simulink model "MPC_fmincon"  (R2023a)
settings: Solver=ode1  StartTime=0.0  StopTime=inf  FixedStep=0.002  RelTol=1e-3  EnableMultiTasking=on
undefined symbols (not defined in the file): HIL
libraries: quarc_library x18, simulink x1
settings Model: ExtModeTrigDuration=10000  Creator=bajdus  LastModifiedBy=pindiche
settings SolverCC: AlgebraicLoopSolver=TrustRegion  PositivePriorityOrder=on
settings DataIOCC: ReturnWorkspaceOutputs=off
settings DebuggingCC: UnconnectedInputMsg=warning  UnconnectedOutputMsg=warning  UnconnectedLineMsg=warning  ArithmeticOperatorsInVariantConditions=warning
settings HardwareCC: ProdBitPerLong=64  ProdLargestAtomicInteger=LongLong  ProdLargestAtomicFloat=Double  ProdLongLongMode=on  ProdHWDeviceType=ARM Compatible->ARM 64-bit (LP64)
settings ModelReferenceCC: EnableRefExpFcnMdlSchedulingChecks=on
settings SFSimCC: SimUseLocalCustomCode=off  CustomCodeUndefinedFunction=UseInterfaceOnly
settings RTWCC: Description=QUARC Linux QCar2 Target Using Toolchain  SystemTargetFile=quarc_linux_qcar2.tlc  TemplateMakefile=quarc_default_tmf  RTWUseLocalCustomCode=off  Toolchain=QUARC linux_qcar2 | gmake (64-bit Windows)  BuildConfiguration=Faster Runs
settings CodeAppCC: StateflowObjectComments=on
settings STFCustomTargetCC: SystemTargetFile=quarc_linux_qcar2.tlc
settings GRTTargetCC: ParMdlRefBuildCompliant=off  CompOptLevelCompliant=off  CombineOutputUpdateFcns=off  MatFileLogging=off  CPPClassGenCompliant=off  GRTInterface=on  ExtMode=on  ExtModeMexFile=quarc_comm  ExtModeMexArgs='-w -d /tmp -uri %u', 'tcpip://192.168.1.126:17001'
settings ConfigComp: CovMetricSettings=dswe

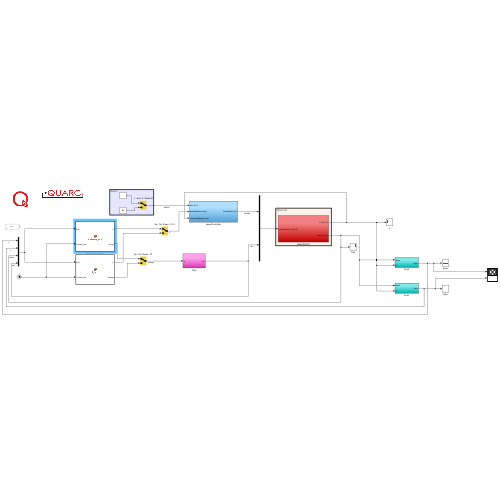
[thumbnail: Simulink's stored preview of the top-level diagram]
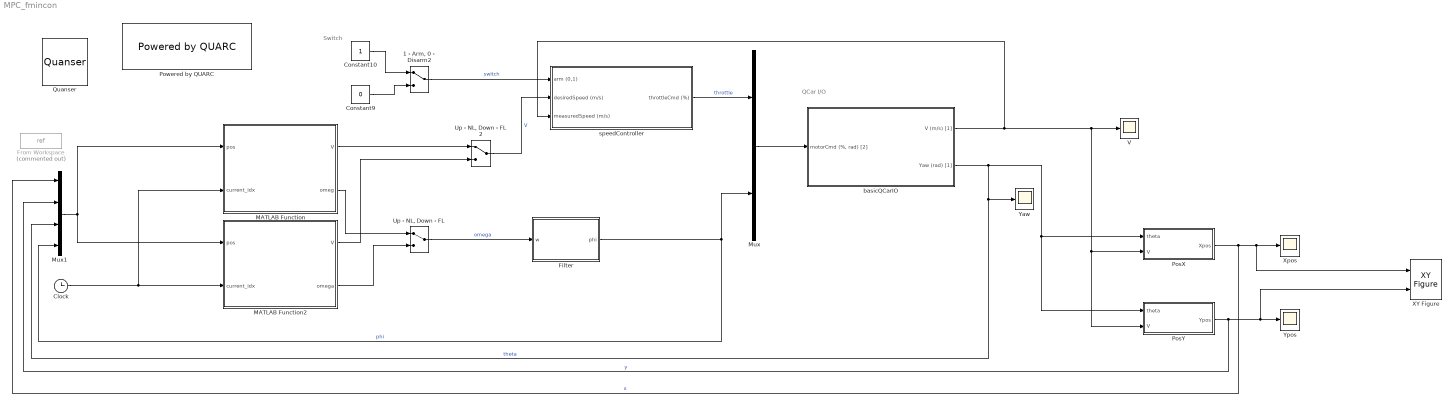
== system MPC_fmincon ==
  note: QCar I/O
  note: Switch
  "1 - Arm, 0 - Disarm2" : ManualSwitch
  Clock : Clock
  Constant10 : Constant
  Constant9 : Constant  Value=0
  Filter : Subsystem
  From Workspace : FromWorkspace  Commented=on  VariableName=ref
  MATLAB Function : MATLAB Function  TreatAsAtomicUnit=on
  MATLAB Function2 : MATLAB Function  TreatAsAtomicUnit=on
  Mux : Mux  Inputs=2
  Mux1 : Mux
  PosX : Subsystem
  PosY : Subsystem
  Powered by QUARC : quarc_library/Logos/Powered by QUARC
  Quanser : quarc_library/Logos/Quanser
  "Up - NL, Down - FL" : ManualSwitch
  "Up - NL, Down - FL 2" : ManualSwitch
  V : Scope
  XY Figure : quarc_library/Sinks/Figures/XY Figure  figure_mode=Use figure window  figure_tag=figure1  axes_tag=axes1  plot_mode=Time-based  minimum_x=-5  maximum_x=5  minimum_y=-5  maximum_y=5  buffer_size=1000000  update_rate=100  initial_position="1.8          41.8         439.2         331.2"  initial_visibility=off  sample_time=-1
      settings: SourceProductName=QUARC Targets
  Xpos : Scope
  Yaw : Scope
  Ypos : Scope
  basicQCarIO : Subsystem
  speedController : Subsystem
  wires:
  Mux/1 -> basicQCarIO/1("motorCmd (%, rad) [2]")
  "1 - Arm, 0 - Disarm2"/1 -> speedController/1(arm (0,1))  "switch"
  Constant10/1 -> "1 - Arm, 0 - Disarm2"/1
  speedController/1(throttleCmd (%)) -> Mux/1  "throttle"
  basicQCarIO/1(V (m/s) [1]) -> speedController/3(measuredSpeed (m/s)), V/1, PosX/2(V), PosY/2(V)
  Constant9/1 -> "1 - Arm, 0 - Disarm2"/2
  PosX/1(Xpos) -> XY Figure/1, Xpos/1, Mux1/1  "x"
  PosY/1(Ypos) -> XY Figure/2, Ypos/1, Mux1/2  "y"
  basicQCarIO/2(Yaw (rad) [1]) -> Mux1/3, Yaw/1, PosY/1(theta), PosX/1(theta)  "theta"
  Filter/1(phi) -> Mux1/4, Mux/2  "phi"
  MATLAB Function/1(V) -> "Up - NL, Down - FL 2"/1
  MATLAB Function2/1(V) -> "Up - NL, Down - FL 2"/2
  "Up - NL, Down - FL 2"/1 -> speedController/2(desiredSpeed (m/s))  "V"
  MATLAB Function/2(omeg) -> "Up - NL, Down - FL"/1
  MATLAB Function2/2(omega) -> "Up - NL, Down - FL"/2
  Mux1/1 -> MATLAB Function/1(pos), MATLAB Function2/1(pos)
  Clock/1 -> MATLAB Function/2(current_idx), MATLAB Function2/2(current_idx)
  "Up - NL, Down - FL"/1 -> Filter/1(w)  "omega"

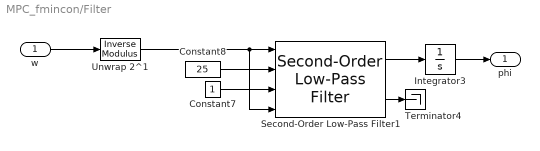
== system MPC_fmincon/Filter ==
  w : Inport
  Constant7 : Constant
  Constant8 : Constant  Value=25
  Integrator3 : Integrator
  Second-Order Low-Pass Filter1 : quarc_library/Continuous/Second-Order Low-Pass Filter  params_source=External (input ports)  input_width=1  input_zeta=1  input_init=0
  Terminator4 : Terminator
  Unwrap 2^1 : quarc_library/Discontinuities/Inverse Modulus  modulus=16777215  output_derivative=off  output_revolutions=off  max_x=Inf  min_x=-Inf
  phi : Outport
  wires:
  Constant8/1 -> Second-Order Low-Pass Filter1/2
  Constant7/1 -> Second-Order Low-Pass Filter1/3
  Second-Order Low-Pass Filter1/1 -> Integrator3/1
  Unwrap 2^1/1 -> Second-Order Low-Pass Filter1/4, Second-Order Low-Pass Filter1/1
  w/1 -> Unwrap 2^1/1
  Second-Order Low-Pass Filter1/2 -> Terminator4/1
  Integrator3/1 -> phi/1

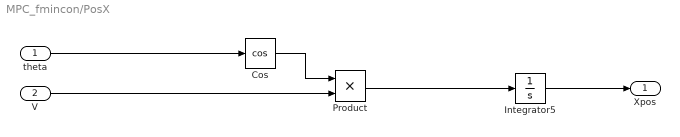
== system MPC_fmincon/PosX ==
  theta : Inport
  V : Inport  Port=2
  Cos : Trigonometry  Operator=cos
  Integrator5 : Integrator
  Product : Product
  Xpos : Outport
  wires:
  Cos/1 -> Product/1
  theta/1 -> Cos/1
  V/1 -> Product/2
  Integrator5/1 -> Xpos/1
  Product/1 -> Integrator5/1

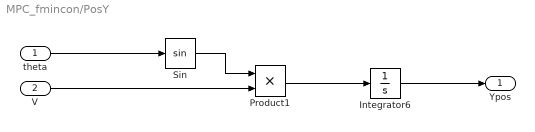
== system MPC_fmincon/PosY ==
  theta : Inport
  V : Inport  Port=2
  Integrator6 : Integrator
  Product1 : Product
  Sin : Trigonometry
  Ypos : Outport
  wires:
  theta/1 -> Sin/1
  V/1 -> Product1/2
  Sin/1 -> Product1/1
  Integrator6/1 -> Ypos/1
  Product1/1 -> Integrator6/1

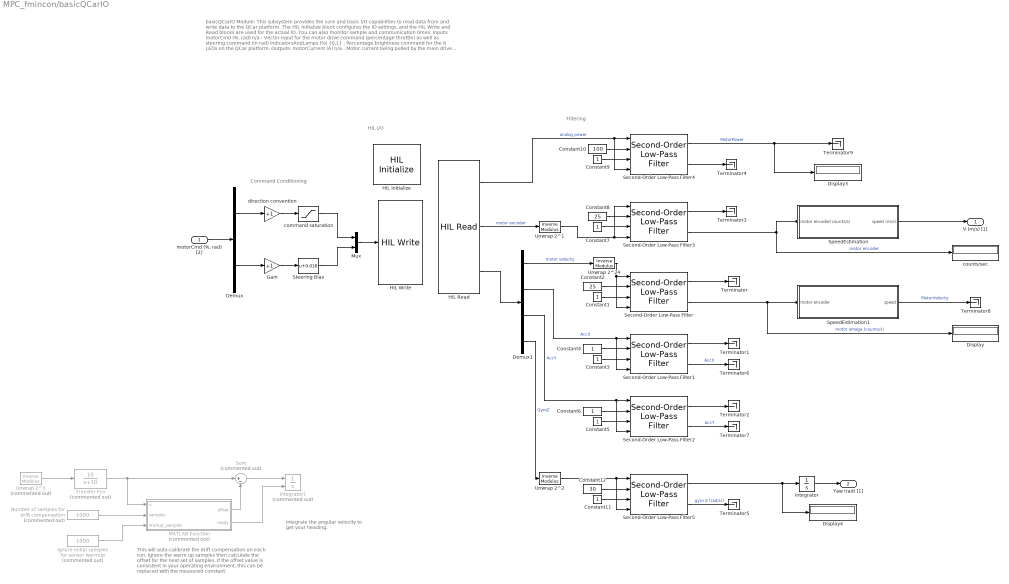
== system MPC_fmincon/basicQCarIO ==
  note: Filtering
  note: basicQCarIO Module:
      |
      | This subsystem provides the core and basic I/O capabilities to read data from and write data to the QCar platform. The HIL Initialize block configures the IO settings, and the HIL Write and Read blocks are used for the actual IO. You can also monitor sample and communication times.
      |
      | Inputs:
      | motorCmd (%, rad) n/a : Vector input for the motor drive command (percentage throttle) as well as steering command (in rad)
      | indicatorsAndLamps (%) {0,1} : Percentage brightness command for the 8 LEDs on the QCar platform.
      |
      | Outputs:
      | motorCurrent (A) n/a : Motor current being pulled by the main drive motor
      | batteryVoltage (V) {0, 12.6} : Current battery voltage reading
      | motorSpeed (counts/s) n/a : Drive motor speed measured using an encoder (do not confuse with wheel speed as this measurement is at the drive shaft)
  note: Command Conditioning
  note: HIL I/O
  note: Integrate the angular velocity to
      | get your heading.
  note: This will auto-calibrate the drift compensation
      | on each run. Ignore the warm up samples
      | then calculate the offset for the next set of samples.
      | If the offset value is consistent in your operating
      | environment, this can be replaced with the measured
      | constant.
  "motorCmd (%, rad) [2]" : Inport
  Constant{1,3..7,9,11} (8 alike) : Constant
  Constant10 : Constant  Value=100
  Constant12 : Constant  Value=30
  Constant2 : Constant  Value=25
  Constant8 : Constant  Value=25
  Demux : Demux  Outputs=2
  Demux1 : Demux
  Display : Display
  Display3 : Display
  Display4 : Display
  Gain : Gain  Gain=+1
  HIL Initialize : quarc_library/Data Acquisition/Generic/Configuration/HIL Initialize  object_name=HIL-2  board_type=qcar2  board_number=0  board_options=gyro_fs=250;gyro_rate=500;gyro_bw=125;gyro_ord=3;accel_fs=16;accel_rate=1000;accel_bw=250;accel_ord=3;temp_bw=4000;enc0_dir=0;enc1_dir=0;enc2_dir=0;steer_bias=0.05;  exclusive=off  active=on  hardware_clocks=[]  clock_modes=[]  initial_clock_frequencies=[]  set_clock_params_at_start=off  set_clock_params_at_switch_in=off  set_clock_frequencies_at_start=off  set_clock_frequencies_at_switch_in=off  analog_input_channels=[0:4]  analog_input_configurations=[]  analog_input_maximums=[3.3]  analog_input_minimums=[0]  set_analog_input_params_at_start=off  set_analog_input_params_at_switch_in=off  analog_output_channels=[]  analog_output_maximums=[]  analog_output_minimums=[]  initial_analog_outputs=[]  final_analog_outputs=[]  watchdog_analog_outputs=[]  set_analog_output_params_at_start=off  set_analog_output_params_at_switch_in=off  set_analog_outputs_at_start=off  set_analog_outputs_at_switch_in=off  set_analog_outputs_at_terminate=off  set_analog_outputs_at_switch_out=off  set_analog_outputs_on_watchdog=off  digital_input_channels=[0:14]  digital_output_channels=[11:26]  digital_output_configuration=[]  initial_digital_outputs=[0]  final_digital_outputs=[0]  watchdog_digital_outputs=[0]  set_digital_output_params_at_start=off  set_digital_output_params_at_switch_in=off  set_digital_outputs_at_start=on  set_digital_outputs_at_switch_in=off  set_digital_outputs_at_terminate=on  set_digital_outputs_at_switch_out=off  set_digital_outputs_on_watchdog=off  encoder_channels=[0:2]  quadrature=[4]  encoder_filter_frequency=100e6/1  initial_encoder_counts=[0]  set_encoder_params_at_start=on  set_encoder_params_at_switch_in=off  set_encoder_counts_at_start=on  set_encoder_counts_at_switch_in=off  pwm_channels=[0:1]  pwm_modes=[0]  pwm_frequency=180e6/4096  pwm_configuration=[0]  pwm_alignment=[0]  pwm_polarity=[1]  pwm_leading_deadband=[]  pwm_trailing_deadband=[]  initial_pwm_outputs=[0]  final_pwm_outputs=[0]  watchdog_pwm_outputs=[0]  set_pwm_params_at_start=on  set_pwm_params_at_switch_in=off  set_pwm_outputs_at_start=on  set_pwm_outputs_at_switch_in=off  set_pwm_outputs_at_terminate=on  set_pwm_outputs_at_switch_out=off  set_pwm_outputs_on_watchdog=off  other_output_channels=[1000 11000]  initial_other_outputs=[0]  final_other_outputs=[0]  watchdog_other_outputs=[0]  set_other_outputs_at_start=on  set_other_outputs_at_switch_in=off  set_other_outputs_at_terminate=on  set_other_outputs_at_switch_out=off  set_other_outputs_on_watchdog=off
  HIL Read : quarc_library/Data Acquisition/Generic/Immediate I//O/HIL Read  object_name=HIL-2  analog_channels=[4]  encoder_channels=[0]  digital_channels=[]  other_channels=[14000 4000:4001 3002]  sample_time=qc_get_step_size  active=on  vector_output=on  data_type_mode=Inherit via back propagation  encoder_data_type=double  digital_data_type=boolean
  HIL Write : quarc_library/Data Acquisition/Generic/Immediate I//O/HIL Write  object_name=HIL-2  analog_channels=[]  pwm_channels=[]  digital_channels=[]  other_channels=[11000 1000]  sample_time=qc_get_step_size  active=off  vector_input=on
  Ignore initial samples for sensor warmup : Constant  Commented=on  Value=1000
  Integrator : Integrator
  Integrator1 : Integrator  Commented=on  ExternalReset=rising
  MATLAB Function : MATLAB Function  Commented=on  TreatAsAtomicUnit=on
  Mux : Mux  Inputs=2
  Number of samples for drift compensation : Constant  Commented=on  Value=1000
  Second-Order Low-Pass Filter{,1..5} (6 alike) : quarc_library/Continuous/Second-Order Low-Pass Filter  params_source=External (input ports)  input_width=1  input_zeta=1  input_init=0
  SpeedEstimation : Subsystem
  SpeedEstimation1 : Subsystem
  Steering Bias : Bias  Bias=0.018  SaturateOnIntegerOverflow=off
  Sum : Sum  Commented=on  Inputs=|+-
  Terminator{,1..9} (10 alike) : Terminator
  Transfer Fcn : TransferFcn  Commented=on  Numerator=[10]  Denominator=[1 10]
  Unwrap 2^1 : quarc_library/Discontinuities/Inverse Modulus  modulus=16777215  output_derivative=off  output_revolutions=off  max_x=Inf  min_x=-Inf
  Unwrap 2^2 : quarc_library/Discontinuities/Inverse Modulus  modulus=16777215  output_derivative=off  output_revolutions=off  max_x=Inf  min_x=-Inf
  Unwrap 2^24 : quarc_library/Discontinuities/Inverse Modulus  modulus=16777215  output_derivative=off  output_revolutions=off  max_x=Inf  min_x=-Inf
  Unwrap 2^3 : quarc_library/Discontinuities/Inverse Modulus  Commented=on  modulus=16777215  output_derivative=off  output_revolutions=off  max_x=Inf  min_x=-Inf
  command saturation : Saturate  UpperLimit=0.25  LowerLimit=-0.25
  counts/sec : Display
  direction convention : Gain  Gain=+1
  V (m/s) [1] : Outport  VectorParamsAs1DForOutWhenUnconnected=off
  Yaw (rad) [1] : Outport  Port=2  VectorParamsAs1DForOutWhenUnconnected=off
  wires:
  Constant2/1 -> Second-Order Low-Pass Filter/2
  Unwrap 2^24/1 -> Second-Order Low-Pass Filter/4, Second-Order Low-Pass Filter/1
  Demux/2 -> Gain/1
  direction convention/1 -> command saturation/1
  "motorCmd (%, rad) [2]"/1 -> Demux/1
  Second-Order Low-Pass Filter/1 -> Terminator/1
  Second-Order Low-Pass Filter/2 -> Display/1, SpeedEstimation1/1(motor encoder)  "motor omega (counts/s)"
  Constant1/1 -> Second-Order Low-Pass Filter/3
  Demux/1 -> direction convention/1
  Gain/1 -> Steering Bias/1
  Constant7/1 -> Second-Order Low-Pass Filter3/3
  Constant8/1 -> Second-Order Low-Pass Filter3/2
  Mux/1 -> HIL Write/1
  command saturation/1 -> Mux/1
  Steering Bias/1 -> Mux/2
  Unwrap 2^1/1 -> Second-Order Low-Pass Filter3/1, Second-Order Low-Pass Filter3/4
  SpeedEstimation/1(speed (m/s)) -> V (m/s) [1]/1
  Demux1/1 -> Unwrap 2^24/1  "motor velocity"
  SpeedEstimation1/1(speed) -> Terminator8/1  "MotorVelocity"
  Second-Order Low-Pass Filter1/1 -> Terminator1/1
  Constant3/1 -> Second-Order Low-Pass Filter1/3
  Constant4/1 -> Second-Order Low-Pass Filter1/2
  Second-Order Low-Pass Filter2/1 -> Terminator2/1
  Constant5/1 -> Second-Order Low-Pass Filter2/3
  Constant6/1 -> Second-Order Low-Pass Filter2/2
  Second-Order Low-Pass Filter2/2 -> Terminator7/1  "AccY"
  Demux1/2 -> Second-Order Low-Pass Filter1/4, Second-Order Low-Pass Filter1/1  "AccX"
  Demux1/3 -> Second-Order Low-Pass Filter2/4, Second-Order Low-Pass Filter2/1  "AccY"
  HIL Read/3 -> Demux1/1
  HIL Read/1 -> Second-Order Low-Pass Filter4/4, Second-Order Low-Pass Filter4/1  "analog power"
  Second-Order Low-Pass Filter4/2 -> Terminator4/1
  Constant9/1 -> Second-Order Low-Pass Filter4/3
  Constant10/1 -> Second-Order Low-Pass Filter4/2
  Second-Order Low-Pass Filter4/1 -> Terminator9/1, Display3/1  "MotorPower"
  Constant12/1 -> Second-Order Low-Pass Filter5/2
  Constant11/1 -> Second-Order Low-Pass Filter5/3
  Second-Order Low-Pass Filter5/2 -> Terminator5/1  "gyro Z (rad/s))"
  Second-Order Low-Pass Filter5/1 -> Display4/1, Integrator/1
  Unwrap 2^2/1 -> Second-Order Low-Pass Filter5/4, Second-Order Low-Pass Filter5/1
  Number of samples for drift compensation/1 -> MATLAB Function/2(samples)
  Ignore initial samples for sensor warmup/1 -> MATLAB Function/3(startup_samples)
  MATLAB Function/1(offset) -> Sum/2
  MATLAB Function/2(ready) -> Integrator1/2
  Sum/1 -> Integrator1/1
  Second-Order Low-Pass Filter3/1 -> Terminator3/1
  Second-Order Low-Pass Filter3/2 -> counts/sec/1, SpeedEstimation/1(motor encoder(counts/s))  "motor encoder"
  Transfer Fcn/1 -> MATLAB Function/1(u), Sum/1
  Unwrap 2^3/1 -> Transfer Fcn/1
  Demux1/4 -> Unwrap 2^2/1  "GyroZ"
  Integrator/1 -> Yaw (rad) [1]/1
  HIL Read/2 -> Unwrap 2^1/1  "motor encoder"
  Second-Order Low-Pass Filter1/2 -> Terminator6/1  "AccX"

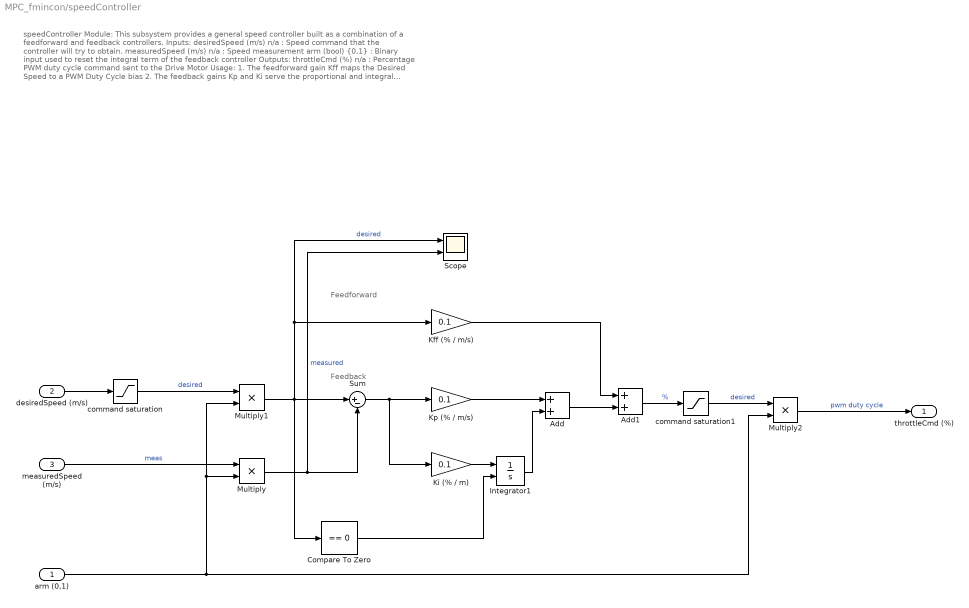
== system MPC_fmincon/speedController ==
  note: Feedforward
  note: Feedback
  note: speedController Module:
      |
      | This subsystem provides a general speed controller built as a combination of a feedforward and feedback controllers.
      |
      | Inputs:
      | desiredSpeed (m/s) n/a : Speed command that the controller will try to obtain.
      | measuredSpeed (m/s) n/a : Speed measurement
      | arm (bool) {0,1} : Binary input used to reset the integral term of the feedback controller
      |
      | Outputs:
      | throttleCmd (%) n/a : Percentage PWM duty cycle command sent to the Drive Motor
      |
      | Usage:
      | 1. The feedforward gain Kff maps the Desired Speed to a PWM Duty Cycle bias
      | 2. The feedback gains Kp and Ki serve the proportional and integral terms to output corrections to the PWM Duty Cycle so as to regulate the desired speed.
  arm (0,1) : Inport
  desiredSpeed (m/s) : Inport  Port=2
  measuredSpeed (m/s) : Inport  Port=3
  Add : Sum
  Add1 : Sum
  Compare To Zero : simulink/Logic and Bit Operations/Compare To Zero  relop===  OutDataTypeStr=boolean
  Integrator1 : Integrator  ExternalReset=either  LimitOutput=on  UpperSaturationLimit=0.4  LowerSaturationLimit=-0.4
  Kff (% / m/s) : Gain  Gain=0.1
  "Ki (% / m) " : Gain  Gain=0.1
  Kp (% / m/s) : Gain  Gain=0.1
  Multiply : Product
  Multiply1 : Product
  Multiply2 : Product
  Scope : Scope  NumInputPorts=2
  Sum : Sum  Inputs=|+-
  command saturation : Saturate  UpperLimit=0.8  LowerLimit=-0.8
  command saturation1 : Saturate
  throttleCmd (%) : Outport  VectorParamsAs1DForOutWhenUnconnected=off
  wires:
  command saturation/1 -> Multiply1/1  "desired"
  arm (0,1)/1 -> Multiply1/2, Multiply/2, Multiply2/2
  measuredSpeed (m/s)/1 -> Multiply/1  "meas"
  Multiply/1 -> Sum/2, Scope/2  "measured"
  Add/1 -> Add1/2
  Multiply1/1 -> Compare To Zero/1, Sum/1, Kff (% / m/s)/1, Scope/1  "desired"
  Integrator1/1 -> Add/2
  Multiply2/1 -> throttleCmd (%)/1  "pwm duty cycle"
  Kp (% / m/s)/1 -> Add/1
  Compare To Zero/1 -> Integrator1/2
  Kff (% / m/s)/1 -> Add1/1
  Sum/1 -> "Ki (% / m) "/1, Kp (% / m/s)/1
  "Ki (% / m) "/1 -> Integrator1/1
  desiredSpeed (m/s)/1 -> command saturation/1
  command saturation1/1 -> Multiply2/1  "desired"
  Add1/1 -> command saturation1/1  "%"

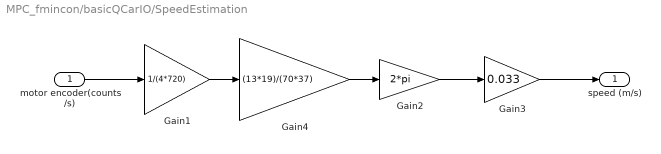
== system MPC_fmincon/basicQCarIO/SpeedEstimation ==
  motor encoder(counts/s) : Inport
  Gain1 : Gain  Gain=1/(4*720)
  Gain2 : Gain  Gain=2*pi
  Gain3 : Gain  Gain=0.033
  Gain4 : Gain  Gain=(13*19)/(70*37)
  speed (m/s) : Outport
  wires:
  motor encoder(counts/s)/1 -> Gain1/1
  Gain1/1 -> Gain4/1
  Gain2/1 -> Gain3/1
  Gain4/1 -> Gain2/1
  Gain3/1 -> speed (m/s)/1

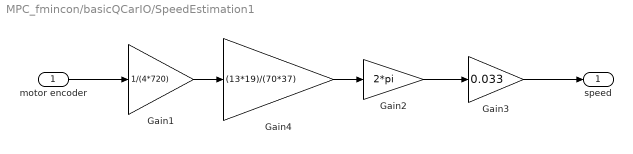
== system MPC_fmincon/basicQCarIO/SpeedEstimation1 ==
  motor encoder : Inport
  Gain1 : Gain  Gain=1/(4*720)
  Gain2 : Gain  Gain=2*pi
  Gain3 : Gain  Gain=0.033
  Gain4 : Gain  Gain=(13*19)/(70*37)
  speed : Outport
  wires:
  motor encoder/1 -> Gain1/1
  Gain1/1 -> Gain4/1
  Gain2/1 -> Gain3/1
  Gain4/1 -> Gain2/1
  Gain3/1 -> speed/1

== matlab function MPC_fmincon/MATLAB Function ==
  data: pos input; current_idx input; V output; omeg output
function [V, omeg] = nonlinear_mpc(pos, current_idx)
    %% Parameters
    Npred = 12;                       
    Q_val = 100; R_val = 3; P_val = 10;
    l = 0.256; Ts = 0.1;
    dx = 4; du = 2;

    % Time
    t = 0 : 0.3 : 10;

    % % % % % % % % % % % % % % % % % 
    % Line reference
    alpha   = 0.3;
    beta    = 0.3;
    xr = alpha * t;     dxr = alpha + 0*t;    ddxr = 0 + 0*t;   dddxr = 0 + 0*t;
    yr = beta * t;      dyr = beta + 0*t;     ddyr = 0 + 0*t;   dddyr = 0 + 0*t;

    % Circle reference
    % alpha   = 1;
    % beta    = 1;
    % ang     = 0.4;
    % xr = alpha*cos(ang*t);      dxr = -alpha*ang*sin(ang*t);    ddxr = -alpha*ang*ang*cos(ang*t);       dddxr = alpha*ang*ang*ang*sin(ang*t);
    % yr = beta*sin(ang*t);       dyr = beta*ang*cos(ang*t);      ddyr = -beta*ang*ang*sin(ang*t);        dddyr = -beta*ang*ang*ang*cos(ang*t);

    % Computing real input reference
    Vr      = sqrt(dxr.*dxr + dyr.*dyr);
    omegar  = l * Vr .* ((dddyr.*dxr - dddxr.*dyr).*Vr.*Vr - 3 * (ddyr.*dxr - ddxr.*dyr) .* (dxr.*ddxr + dyr.*ddyr)) ...
              ./ (Vr.^6 + l*l*(ddyr.*dxr - ddxr.*dyr).^2);
    uref = [Vr; omegar];

    % Computing angle reference
    thetar  = unwrap(atan2(dyr ./ Vr, dxr ./ Vr));
    phir    = atan((l*(ddyr.*dxr - ddxr.*dyr)) ./ Vr.^3);

    xref = [xr; yr; thetar; phir];

    xref_traj = xref;
    uref_traj = uref;

    % Input constraints
    Vmin = -1; Vmax = 1;
    omegamin = -0.8; omegamax = 0.8;

    % State constraint (steering angle phi)
    phimax = pi/5;

    % Weights
    Q = Q_val * eye(dx); Q(3,3) = 10; Q(4,4) = 5;
    R = R_val * eye(du);
    P = P_val * Q;

    % Time horizon check
    T = size(xref_traj, 2);
    horizon_idx = current_idx : min(current_idx + Npred, T);
    horizon_idx = mod(current_idx : current_idx + Npred - 1, T) + 1;
    N = length(horizon_idx);  % Adjust prediction length if close to end

    % Extract horizon reference slices
    xref = xref_traj(:, horizon_idx);
    uref = uref_traj(:, horizon_idx);

    % Initial state
    x0 = pos(:);

    % Initial guess
    u0 = zeros(du * N, 1);

    % Input bounds
    lb = repmat([Vmin; omegamin], N, 1);
    ub = repmat([Vmax; omegamax], N, 1);

    % Solver options
    options = optimoptions('fmincon', ...
        'Display', 'off', ...
        'Algorithm', 'sqp', ...
        'MaxIterations', 100);

    % Objective & constraints
    costfun = @(u) objective_function(u, x0, xref, uref, N, Ts, Q, R, P, l);
    nonlcon = @(u) dynamics_constraints(u, x0, N, Ts, l, phimax);

    % Solve optimization
    u_opt = fmincon(costfun, u0, [], [], [], [], lb, ub, nonlcon, options);

    % Return first control input
    V = u_opt(1);
    omeg = u_opt(2);
end

function J = objective_function(u, x0, xref, uref, N, Ts, Q, R, P, l)
    dx = length(x0); du = 2;
    x = zeros(dx, N+1);
    x(:,1) = x0;
    J = 0;

    for k = 1:N
        u_k = u((k-1)*du+1 : k*du);
        x(:,k+1) = x(:,k) + Ts * vehicle_dynamics(x(:,k), u_k, l);

        err_x = x(:,k) - xref(:,k);
        err_u = u_k - uref(:,k);
        J = J + err_x' * Q * err_x + err_u' * R * err_u;
    end

    err_final = x(:,end) - xref(:,end);
    J = J + err_final' * P * err_final;
end


function [c, ceq] = dynamics_constraints(u, x0, N, Ts, l, phimax)
    dx = length(x0); du = 2;
    x = zeros(dx, N+1);
    x(:,1) = x0;
    ceq = [];

    for k = 1:N
        u_k = u((k-1)*du+1 : k*du);
        x_next = x(:,k) + Ts * vehicle_dynamics(x(:,k), u_k, l);
        x(:,k+1) = x_next;
        ceq = [ceq; x(:,k+1) - x_next];
    end

    % Inequality: -phimax ≤ phi_k ≤ phimax
    phi = x(4,2:end); % skip initial phi
    c = [phi' - phimax;
        -phi' - phimax];
end

function dxdt = vehicle_dynamics(x, u, l)
    dxdt = [u(1) * cos(x(3));
            u(1) * sin(x(3));
            u(1)/l * tan(x(4));
            u(2)];
end

== matlab function MPC_fmincon/basicQCarIO/MATLAB Function ==
  settings: updateMethod=DISCRETE
  data: u input; offset output; samples input; ready output; startup_samples input
function [offset, ready] = fcn(u, samples, startup_samples)

persistent sample_sum;
persistent remaining_samples;
persistent last_offset;
persistent last_ready;
persistent remaining_startup_samples;

if isempty(sample_sum)
    sample_sum = 0;
    remaining_samples = samples;
    remaining_startup_samples = startup_samples;
    last_offset = 0;
    last_ready = 0;
end

if (remaining_startup_samples > 0)
    remaining_startup_samples = remaining_startup_samples - 1;
else
    if (remaining_samples > 0) && (samples > 0)
        sample_sum = sample_sum + u;
        remaining_samples = remaining_samples - 1;

        if remaining_samples == 0
            last_offset = sample_sum/samples;
            last_ready = 1;
        end
    end
end

offset = last_offset;
ready = last_ready;

== matlab function MPC_fmincon/MATLAB Function2 ==
  data: pos input; V output; current_idx input; omega output
function [V, omega] = fl_mpc(pos, current_idx)    
    %% Parameters
    Npred = 5;                       
    Q_val = 10; R_val = 1; P_val = 1;
    l = 0.256; Ts = 0.3;
    Delta = 0.35; 
    dx = 4; du = 2; dz = 2;

    % Time
    t = 0:0.5:10;   % Adjusted to end when distance = 0.5 meters
    
    % Straight line along X direction
    alpha = 0.2;       % constant speed in m/s
    beta = 0.2;
    xr = alpha * t;     % x increases linearly
    yr = beta * t;  % y remains constant

    % Derivatives
    dxr = alpha * ones(size(t));
    dyr = beta * ones(size(t));

    ddxr = zeros(size(t));
    ddyr = zeros(size(t));

    dddxr = zeros(size(t));
    dddyr = zeros(size(t));

    % Computing real input reference
    Vr      = sqrt(dxr.*dxr + dyr.*dyr);
    omegar  = l * Vr .* ((dddyr.*dxr - dddxr.*dyr).*Vr.*Vr - 3 * (ddyr.*dxr - ddxr.*dyr) .* (dxr.*ddxr + dyr.*ddyr)) ...
              ./ (Vr.^6 + l*l*(ddyr.*dxr - ddxr.*dyr).^2);

    % Computing angle reference
    thetar  = unwrap(atan2(dyr ./ Vr, dxr ./ Vr));
    phir    = atan((l*(ddyr.*dxr - ddxr.*dyr)) ./ Vr.^3);

    uref = [Vr; omegar];
    xref = [xr; yr; thetar; phir];

    % Computing references on z and virtual input w
    zref = [xr + l*cos(thetar) + Delta*cos(thetar + phir);
            yr + l*sin(thetar) + Delta*sin(thetar + phir)];
    
    etaref = [thetar; phir];
    
    wref = zeros(2, numel(t));
    len = numel(t);
    wref = zeros(2, length(xr));
    len = length(xr);
    for i = 1:len
        s1        = sin(thetar(i) + phir(i)); 
        c1        = cos(thetar(i) + phir(i));
        M         = [cos(thetar(i)) - tan(phir(i))*(sin(thetar(i)) + Delta*s1/l), -Delta*s1;
                     sin(thetar(i)) + tan(phir(i))*(cos(thetar(i)) + Delta*c1/l),  Delta*c1];
        wref(:,i) = M * uref(:,i);
    end

    zref_traj = zref;
    wref_traj = wref;

   %% Constraints
    rhat = min(Delta*l*10/sqrt(Delta*Delta + l*l), 0.5);
    
    % Weights for cost function
    Q = Q_val * eye(dz);
    R = R_val * eye(du);
    P = P_val * Q;
    A = eye(dz);
    B = Ts * eye(dz);

    % Time horizon check
    T = size(zref_traj, 2);
    horizon_idx = current_idx : min(current_idx + Npred, T);
    N = length(horizon_idx);  % Adjust prediction length if close to end

    % Extract horizon reference slices
    zref = zref_traj(:, horizon_idx);
    wref = wref_traj(:, horizon_idx);

    % Initial state
    x0 = pos(:);

    % Initial guess
    u0 = zeros(du * N, 1);

    % Input bounds
    % lb = repmat([Vmin; omegamin], N, 1);
    % ub = repmat([Vmax; omegamax], N, 1);
    lb = [];
    ub = [];

    % Solver options
    options = optimoptions('fmincon', ...
        'Display', 'off', ...
        'Algorithm', 'sqp', ...
        'MaxIterations', 100);

    % Objective & constraints
    costfun = @(w) objective_function(w, x0, zref, wref, N, Ts, Q, R, P, A, B, Delta, l);
    nonlcon = @(w) dynamics_constraints(w, x0, N, Ts, Delta, l, A, B, rhat);

    % Solve optimization
    w_opt = fmincon(costfun, u0, [], [], [], [], lb, ub, nonlcon, options);
    
    % phi0 = atan2(w_opt(2), w_opt(1));
    M = LinMatrix(x0(3), x0(4), Delta, l);
    u_opt = M^(-1) * w_opt(1:2);

    % Return first control input
    V = u_opt(1);
    omega = u_opt(2);
end

function z = LinOutput(q,phi,Delta,L)
z = [q(1)+L*cos(q(3))+Delta*cos(q(3)+phi);
     q(2)+L*sin(q(3))+Delta*sin(q(3)+phi)];
end

function M = LinMatrix(theta, phi, Delta, L)
s1 = sin(theta+phi); c1 = cos(theta+phi); 
M = [cos(theta)-tan(phi)*(sin(theta)+Delta*s1/L), -Delta*s1;
     sin(theta)+tan(phi)*(cos(theta)+Delta*c1/L),  Delta*c1];
end

function O = LinDyna(eta,L,Delta)
s1 = sin(eta(1)+eta(2)); c1 = cos(eta(1)+eta(2)); 
O = [sin(eta(2))*c1/L,             sin(eta(2))*s1/L;
    -sin(eta(2))*c1/L-s1/Delta,    -sin(eta(2))*s1/L-c1/Delta];
end


function J = objective_function(w, x0, zref, wref, N, Ts, Q, R, P, A, B, Delta, l)
    dz = 2; du = 2;
    z = zeros(dz, N+1);
    phi0 = atan2(w(2), w(1));
    z(:,1) = LinOutput(x0, x0(4), Delta, l);
    J = 0;

    for k = 1:N
        w_k = w((k-1)*du+1 : k*du);
        z(:, k+1) = A * z(:,k) + B * w_k;

        err_z = z(:,k) - zref(:,k);
        err_w = w_k - wref(:,k);
        J = J + err_z' * Q * err_z + err_w' * R * err_w;
    end

    err_final = z(:,end) - zref(:,end);
    J = J + err_final' * P * err_final;
end


function [c, ceq] = dynamics_constraints(w, x0, N, Ts, Delta, l, A, B, rhat)
    dz = 2; du = 2;
    z = zeros(dz, N+1);
    eta = zeros(dz, N+1);
    phi0 = atan2(w(2), w(1));
    z(:,1) = LinOutput(x0, x0(4), Delta, l);
    eta(:,1) = [x0(3); phi0];
    ceq = [];
    c = [];

    for k = 1:N
        w_k = w((k-1)*du+1 : k*du);
        z_next = A * z(:, k) + B * w_k;
        z(:,k+1) = z_next;
        
        O = LinDyna(eta(:, k), l, Delta);
        eta_next = eta(:,k) + Ts * O * w_k;
        eta(:,k+1) = eta_next;
        
        ceq = [ceq; z(:,k+1) - z_next; eta(:,k+1) - eta_next];
        c = [c; w_k' * w_k - rhat];
    end

end

function dxdt = vehicle_dynamics(x, u, l)
    dxdt = [u(1) * cos(x(3));
            u(1) * sin(x(3));
            u(1)/l * tan(x(4));
            u(2)];
end
